simulink model "Smith"  (R2019a)
settings: Solver=FixedStepAuto  StartTime=0.0  StopTime=1200  FixedStep=0.001  RelTol=1e-3
settings Model: Creator=melol  LastModifiedBy=guima

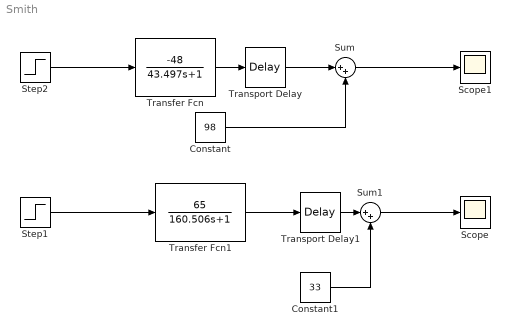
== system Smith ==
  Constant : Constant  Value=98
  Constant1 : Constant  Value=33
  Scope : Scope
  Scope1 : Scope
  Step1 : Step  Time=0  SampleTime=0
  Step2 : Step  Time=0  SampleTime=0
  Sum : Sum  Inputs=|++
  Sum1 : Sum  Inputs=|++
  Transfer Fcn : TransferFcn  Numerator=[-48]  Denominator=[43.497 1]
  Transfer Fcn1 : TransferFcn  Numerator=[65]  Denominator=[160.506 1]
  Transport Delay : TransportDelay  DelayTime=17.502
  Transport Delay1 : TransportDelay  DelayTime=0
  wires:
  Transfer Fcn1/1 -> Transport Delay1/1
  Step1/1 -> Transfer Fcn1/1
  Step2/1 -> Transfer Fcn/1
  Constant/1 -> Sum/2
  Transfer Fcn/1 -> Transport Delay/1
  Transport Delay/1 -> Sum/1
  Transport Delay1/1 -> Sum1/1
  Constant1/1 -> Sum1/2
  Sum/1 -> Scope1/1
  Sum1/1 -> Scope/1
